simulink model "zoh"  (R2015b)
settings: Solver=VariableStepAuto  StartTime=0.0  StopTime=1/200  RelTol=1e-3
settings Model: Creator=ovi  LastModifiedBy=ovi

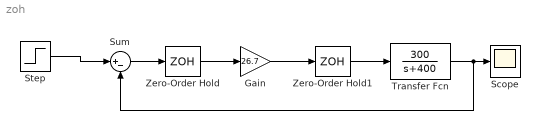
== system zoh ==
  Gain : Gain  Gain=26.7
  Scope : Scope
  Step : Step  Time=0  SampleTime=0
  Sum : Sum  Inputs=|+-
  Transfer Fcn : TransferFcn  Numerator=[300]  Denominator=[1 400]
  Zero-Order Hold : ZeroOrderHold  SampleTime=1/400/10
  Zero-Order Hold1 : ZeroOrderHold  SampleTime=1/400/10
  wires:
  Transfer Fcn/1 -> Sum/2, Scope/1
  Zero-Order Hold/1 -> Gain/1
  Sum/1 -> Zero-Order Hold/1
  Step/1 -> Sum/1
  Gain/1 -> Zero-Order Hold1/1
  Zero-Order Hold1/1 -> Transfer Fcn/1
